simulink subsystem "VCM_main_djustablegain"  (R2021b)
settings: Solver=VariableStepAuto  StartTime=0.0  StopTime=10.0  RelTol=1e-3
undefined symbols (not defined in the file): df, dr, g, gear_f, gear_r, Iwf, Iwr, l, lf, M, Rwf, Rwr
libraries: simulink x43, dspstat3 x2, dspswit3 x1
(part 3 of 3)

== system VCM_main_djustablegain/VDC/Launch/max rpm ==
  Can Inv : Inport
  Bus Selector4 : BusSelector  OutputSignals=MC_11.MC1_Actual speed value in 1/rpm,MC_31.MC3_Actual speed value in 1/rpm,MC_21.MC2_Actual speed value in 1/rpm,MC_41.MC4_Actual speed value in 1/rpm
  Min : MinMax  Function=max  Inputs=4
  max rpm : Outport
  wires:
  Bus Selector4/2 -> Min/2  "<MC3_Actual speed value in 1/rpm>"
  Bus Selector4/3 -> Min/3  "<MC2_Actual speed value in 1/rpm>"
  Bus Selector4/1 -> Min/1  "<MC1_Actual speed value in 1/rpm>"
  Min/1 -> max rpm/1  "max rpm"
  Can Inv/1 -> Bus Selector4/1
  Bus Selector4/4 -> Min/4  "<MC4_Actual speed value in 1/rpm>"

== system VCM_main_djustablegain/VDC/Torque Front//rear distributor Main/Max Torque Limit ==
  note: MAXトルクオーバーしている分だけもう一方に振り直し
  Max Torque : Inport
  torque_front : Inport  Port=2
  torque_rear : Inport  Port=3
  Add10 : Sum  Inputs=-+
  Add11 : Sum
  Add4 : Sum  Inputs=+-
  Add7 : Sum  Inputs=+-
  Add8 : Sum
  Add9 : Sum  Inputs=+-
  Display : Display
  Display5 : Display
  Display6 : Display
  Saturation : Saturate  UpperLimit=inf  LowerLimit=0
  Saturation3 : Saturate  UpperLimit=inf  LowerLimit=0
  torque_front Out : Outport
  torque_rear Out : Outport  Port=2
  wires:
  Max Torque/1 -> Add9/2, Add4/2
  Add11/1 -> torque_rear Out/1
  Add7/1 -> Add11/2
  Add4/1 -> Saturation/1
  Add10/1 -> torque_front Out/1
  Add8/1 -> Add10/2
  torque_rear/1 -> Display6/1, Add7/1, Add4/1
  Add9/1 -> Saturation3/1
  torque_front/1 -> Display5/1, Add8/1, Add9/1
  Saturation3/1 -> Add10/1, Add11/1
  Saturation/1 -> Display/1, Add7/2, Add8/2

== system VCM_main_djustablegain/VDC/Torque Front//rear distributor Main/Min Torque Limit ==
  note: MINトルクオーバーしている分だけもう一方に振り直し
  Min Torque : Inport
  torque_front : Inport  Port=2
  torque_rear : Inport  Port=3
  Add10 : Sum  Inputs=-+
  Add11 : Sum
  Add4 : Sum  Inputs=+-
  Add7 : Sum  Inputs=+-
  Add8 : Sum
  Add9 : Sum  Inputs=+-
  Display{,1..2,5..6} (5 alike) : Display
  Gain : Gain  Gain=-1
  Saturation : Saturate  UpperLimit=0  LowerLimit=-inf
  Saturation3 : Saturate  UpperLimit=0  LowerLimit=-inf
  torque_rear Out : Outport
  torque_front Out : Outport  Port=2
  wires:
  Gain/1 -> Add9/2, Add4/2
  Min Torque/1 -> Gain/1
  Add11/1 -> torque_rear Out/1  "torque_rear"
  Add7/1 -> Add11/2, Display1/1
  Add4/1 -> Saturation/1
  Add10/1 -> torque_front Out/1  "torque_front"
  Add8/1 -> Add10/2
  torque_rear/1 -> Display6/1, Add7/1, Add4/1
  Add9/1 -> Saturation3/1
  torque_front/1 -> Display5/1, Add8/1, Add9/1
  Saturation3/1 -> Add10/1, Add11/1, Display2/1
  Saturation/1 -> Display/1, Add7/2, Add8/2

== system VCM_main_djustablegain/VDC/Torque Front//rear distributor Main/Saturation ==
  u : Inport
  Saturation Dynamic1 : simulink/Discontinuities/Saturation Dynamic  OutMin=[]  OutMax=[]  OutDataTypeStr=Inherit: Same as second input  OutDataType=fixdt(1, 16)  OutScaling=2^-10  DoSatur=off
  y : Outport
  wires:
  [MinTorque] -> Saturation Dynamic1/3
  u/1 -> Saturation Dynamic1/2
  Saturation Dynamic1/1 -> y/1
  [MaxTorque] -> Saturation Dynamic1/1

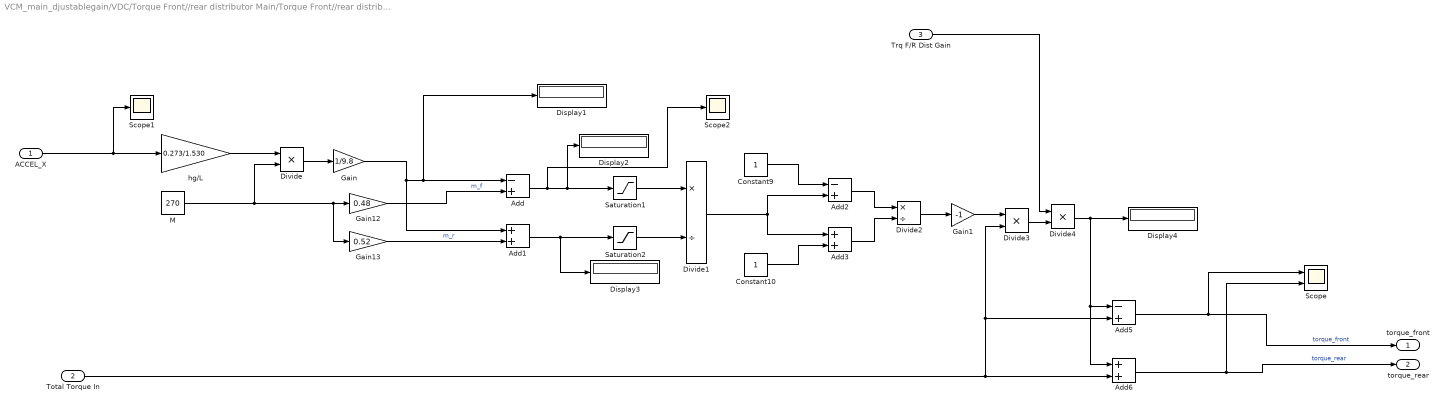
== system VCM_main_djustablegain/VDC/Torque Front//rear distributor Main/Torque Front//rear distributor  ==
  ACCEL_X : Inport
  Total Torque In : Inport  Port=2
  Trq F/R Dist Gain : Inport  Port=3
  Add : Sum  Inputs=-+
  Add1 : Sum
  Add2 : Sum  Inputs=-+
  Add3 : Sum
  Add5 : Sum  Inputs=-+
  Add6 : Sum
  Constant10 : Constant
  Constant9 : Constant
  Display{1..4} (4 alike) : Display
  Divide : Product  Inputs=**
  Divide1 : Product  Inputs=*/
  Divide2 : Product  Inputs=*/
  Divide3 : Product  Inputs=**
  Divide4 : Product  Inputs=**
  Gain : Gain  Gain=1/9.8
  Gain1 : Gain  Gain=-1
  Gain12 : Gain  Gain=0.48
  Gain13 : Gain  Gain=0.52
  M : Constant  Value=270
  Saturation1 : Saturate  UpperLimit=270  LowerLimit=10
  Saturation2 : Saturate  UpperLimit=270  LowerLimit=10
  Scope : Scope  NumInputPorts=2
  Scope1 : Scope
  Scope2 : Scope
  hg/L : Gain  Gain=0.273/1.530
  torque_front : Outport
  torque_rear : Outport  Port=2
  wires:
  Divide/1 -> Gain/1
  Total Torque In/1 -> Divide3/2, Add5/2, Add6/2
  Trq F/R Dist Gain/1 -> Divide4/1
  Divide3/1 -> Divide4/2
  Add5/1 -> torque_front/1, Scope/1  "torque_front"
  Add6/1 -> torque_rear/1, Scope/2  "torque_rear"
  Gain13/1 -> Add1/2  "m_r"
  Saturation1/1 -> Divide1/1
  Add/1 -> Saturation1/1, Display2/1, Scope2/1
  Gain/1 -> Add/1, Display1/1, Add1/1
  Add1/1 -> Saturation2/1, Display3/1
  ACCEL_X/1 -> hg/L/1, Scope1/1
  hg/L/1 -> Divide/1
  Constant10/1 -> Add3/2
  Gain1/1 -> Divide3/1
  Add2/1 -> Divide2/1
  Gain12/1 -> Add/2  "m_f"
  Divide2/1 -> Gain1/1
  Constant9/1 -> Add2/1
  Saturation2/1 -> Divide1/2
  Divide4/1 -> Display4/1, Add5/1, Add6/1
  Add3/1 -> Divide2/2
  Divide1/1 -> Add2/2, Add3/1
  M/1 -> Gain12/1, Gain13/1, Divide/2

== system VCM_main_djustablegain/VDC/Traction Control/Acc Estimater ==
  1/Gear{1..4} (4 alike) : Gain  Gain=gear_r
  Add : Sum  Inputs=++++
  EstLongAcc1 : Scope
  Gain : Gain  Gain=1/(M+2*Iwf/Rwf/Rwf+2*Iwr/Rwr/Rwr)
  Gain1 : Gain  Gain=1/g
  Moving Average : dspstat3/Moving Average  Method=Sliding window  ForgettingFactorPort=off  SpecifyWindowLength=on  WindowLength=10  ForgettingFactor=0.9  SimulateUsing=Code generation
  Rtire{1..4} (4 alike) : Gain  Gain=1/Rwf
  Saturation : Saturate  UpperLimit=1.3*g  LowerLimit=-1.3*g
  EstLongAcc : Outport
  wires:
  [FL_Torque] -> 1/Gear2/1
  Gain/1 -> Moving Average/1  "LongAcc"
  Rtire1/1 -> Add/1
  [RL_Torque] -> 1/Gear4/1
  Rtire3/1 -> Add/3
  1/Gear3/1 -> Rtire4/1
  [FR_Torque] -> 1/Gear1/1
  1/Gear2/1 -> Rtire1/1
  Saturation/1 -> EstLongAcc/1, Gain1/1  "LongAcc"
  Rtire2/1 -> Add/2
  Add/1 -> Gain/1
  1/Gear1/1 -> Rtire2/1
  Gain1/1 -> EstLongAcc1/1
  Rtire4/1 -> Add/4
  1/Gear4/1 -> Rtire3/1
  Moving Average/1 -> Saturation/1
  [RR_Torque] -> 1/Gear3/1

== system VCM_main_djustablegain/VDC/Traction Control/ActualSpeed ==
  Bus Creator : BusCreator  Inputs=4
  ActualSpeed : Outport
  wires:
  [RL_ActualSpeed] -> Bus Creator/3  "RL"
  [FR_ActualSpeed] -> Bus Creator/2  "FR"
  [FL_ActualSpeed] -> Bus Creator/1  "FL"
  [RR_ActualSpeed] -> Bus Creator/4  "RR"
  Bus Creator/1 -> ActualSpeed/1  "ActualSpeed"

== system VCM_main_djustablegain/VDC/Traction Control/Fx Estimater ==
  Bus Creator : BusCreator  Inputs=4
  EstFx : Scope
  FxEstimater : Subsystem
  FxEstimater1 : Subsystem
  FxEstimater2 : Subsystem
  FxEstimater3 : Subsystem
  Fx : Outport
  wires:
  FxEstimater1/1(Fx) -> Bus Creator/2  "FR"
  Bus Creator/1 -> Fx/1, EstFx/1  "Fx"
  FxEstimater3/1(Fx) -> Bus Creator/4  "RR"
  FxEstimater2/1(Fx) -> Bus Creator/3  "RL"
  FxEstimater/1(Fx) -> Bus Creator/1  "FL"
  [FL_Torque] -> FxEstimater/1(Torque)
  [FL_ActualSpeed] -> FxEstimater/2(ActualSpeed)
  [FR_ActualSpeed] -> FxEstimater1/2(ActualSpeed)
  [FR_Torque] -> FxEstimater1/1(Torque)
  [RR_Torque] -> FxEstimater3/1(Torque)
  [RR_ActualSpeed] -> FxEstimater3/2(ActualSpeed)
  [RL_ActualSpeed] -> FxEstimater2/2(ActualSpeed)
  [RL_Torque] -> FxEstimater2/1(Torque)

== system VCM_main_djustablegain/VDC/Traction Control/Load Estimater ==
  Long Acc : Inport
  Sensor : Inport  Port=2
  Steer : Inport  Port=3
  Bus Creator : BusCreator  Inputs=4
  Bus Selector : BusSelector  OutputSignals=CAN_from_IMU_139.VELOCITY_X
  Bus Selector1 : BusSelector  OutputSignals=CAN_from_IMU_121.ACCEL_Y
  Constant : Constant  Value=l
  Divide : Product  Inputs=*/
  Divide1 : Product  Inputs=*/
  EstAcc : Scope  NumInputPorts=2
  EstLoad : Scope
  FR Load Diff : Subsystem  ReferencedSubsystem=FR_Load_Diff
  Gain : Gain  Gain=1/(2*pi)
  Off : Gain  Gain=0
  Product : Product
  RL Load Diff : Subsystem  ReferencedSubsystem=RL_Load_Diff
  Load : Outport
  wires:
  Constant/1 -> Divide/1
  Divide/1 -> Divide1/2  "R"
  RL Load Diff/4 -> Bus Creator/4  "RR"
  Divide1/1 -> EstAcc/2
  Steer/1 -> Gain/1
  RL Load Diff/1 -> Bus Creator/1  "FL"
  FR Load Diff/1 -> RL Load Diff/1  "FrontLoad"
  Bus Selector1/1 -> Off/1  "<ACCEL_Y>"
  FR Load Diff/2 -> RL Load Diff/2  "RearLoad"
  RL Load Diff/2 -> Bus Creator/2  "FR"
  Long Acc/1 -> FR Load Diff/1, EstAcc/1
  RL Load Diff/3 -> Bus Creator/3  "RL"
  Gain/1 -> Divide/2
  Off/1 -> RL Load Diff/3
  Bus Creator/1 -> Load/1, EstLoad/1  "Load"
  Sensor/1 -> Bus Selector1/1, Bus Selector/1
  Bus Selector/1 -> Product/1, Product/2  "<VELOCITY_X>"
  Product/1 -> Divide1/1

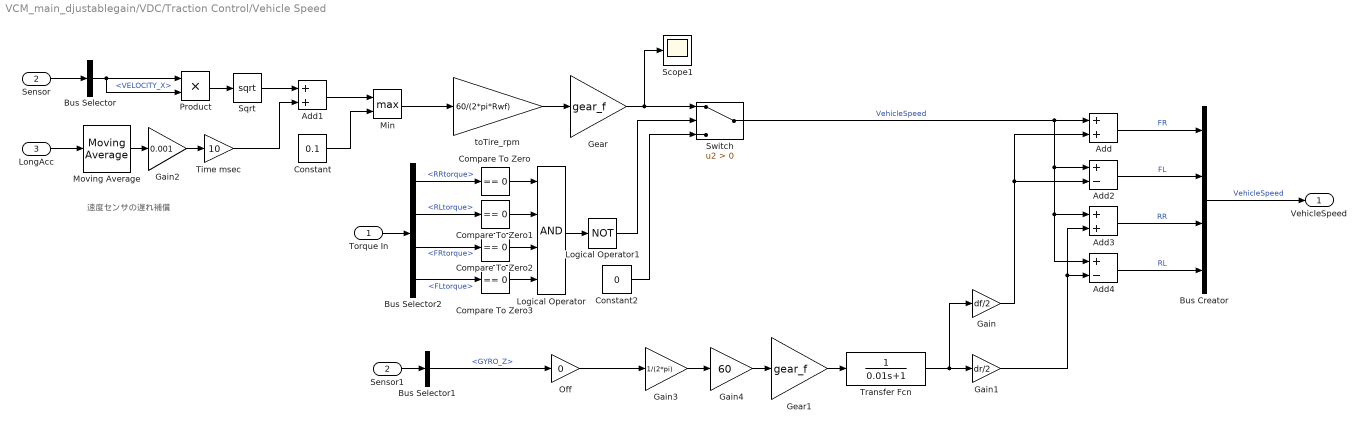
== system VCM_main_djustablegain/VDC/Traction Control/Vehicle Speed ==
  note: 速度センサの遅れ補償
  Torque In : Inport
  Sensor : Inport  Port=2
  LongAcc : Inport  Port=3
  Add : Sum
  Add1 : Sum
  Add2 : Sum  Inputs=+-
  Add3 : Sum
  Add4 : Sum  Inputs=+-
  Bus Creator : BusCreator  Inputs=4
  Bus Selector : BusSelector  OutputSignals=CAN_from_IMU_139.VELOCITY_X
  Bus Selector1 : BusSelector  OutputSignals=CAN_from_IMU_122.GYRO_Z
  Bus Selector2 : BusSelector  OutputSignals=RRtorque,RLtorque,FRtorque,FLtorque
  Compare To Zero{,1..3} (4 alike) : simulink/Logic and Bit Operations/Compare To Zero  relop===  OutDataTypeStr=boolean
  Constant : Constant  Value=0.1
  Constant2 : Constant  Value=0
  Gain : Gain  Gain=df/2
  Gain1 : Gain  Gain=dr/2
  Gain2 : Gain  Gain=0.001
  Gain3 : Gain  Gain=1/(2*pi)
  Gain4 : Gain  Gain=60
  Gear : Gain  Gain=gear_f
  Gear1 : Gain  Gain=gear_f
  Logical Operator : Logic  Inputs=4  AllPortsSameDT=off  OutDataTypeStr=boolean
  Logical Operator1 : Logic  Operator=NOT  AllPortsSameDT=off  OutDataTypeStr=boolean
  Min : MinMax  Function=max  Inputs=2
  Moving Average : dspstat3/Moving Average  Method=Sliding window  ForgettingFactorPort=off  SpecifyWindowLength=on  WindowLength=80  ForgettingFactor=0.9  SimulateUsing=Code generation
  Off : Gain  Gain=0
  Product : Product
  Scope1 : Scope
  Sensor1 : InportShadow  Port=2
  Sqrt : Sqrt  SaturateOnIntegerOverflow=on
  Switch : Switch  Criteria=u2 > Threshold
  Time msec : Gain  Gain=10
  Transfer Fcn : TransferFcn  Denominator=[0.01 1]
  toTire_rpm : Gain  Gain=60/(2*pi*Rwf)
  VehicleSpeed : Outport
  wires:
  Gain3/1 -> Gain4/1
  Bus Selector1/1 -> Off/1  "<GYRO_Z>"
  Product/1 -> Sqrt/1
  Transfer Fcn/1 -> Gain1/1, Gain/1
  Bus Selector/1 -> Product/1, Product/2  "<VELOCITY_X>"
  Switch/1 -> Add/1, Add2/1, Add4/1, Add3/1  "VehicleSpeed"
  Compare To Zero/1 -> Logical Operator/1
  Sensor/1 -> Bus Selector/1
  Bus Selector2/4 -> Compare To Zero3/1  "<FLtorque>"
  Compare To Zero2/1 -> Logical Operator/3
  Torque In/1 -> Bus Selector2/1
  LongAcc/1 -> Moving Average/1
  Sqrt/1 -> Add1/1
  Gear/1 -> Scope1/1, Switch/1
  toTire_rpm/1 -> Gear/1
  Gain1/1 -> Add3/2, Add4/2
  Logical Operator/1 -> Logical Operator1/1
  Add3/1 -> Bus Creator/3  "RR"
  Bus Selector2/1 -> Compare To Zero/1  "<RRtorque>"
  Logical Operator1/1 -> Switch/2
  Sensor1/1 -> Bus Selector1/1
  Compare To Zero3/1 -> Logical Operator/4
  Constant/1 -> Min/2
  Bus Selector2/2 -> Compare To Zero1/1  "<RLtorque>"
  Time msec/1 -> Add1/2
  Bus Selector2/3 -> Compare To Zero2/1  "<FRtorque>"
  Compare To Zero1/1 -> Logical Operator/2
  Off/1 -> Gain3/1
  Constant2/1 -> Switch/3
  Min/1 -> toTire_rpm/1
  Gain/1 -> Add/2, Add2/2
  Add1/1 -> Min/1
  Add2/1 -> Bus Creator/2  "FL"
  Moving Average/1 -> Gain2/1
  Add/1 -> Bus Creator/1  "FR"
  Add4/1 -> Bus Creator/4  "RL"
  Gain2/1 -> Time msec/1
  Gain4/1 -> Gear1/1
  Bus Creator/1 -> VehicleSpeed/1  "VehicleSpeed"
  Gear1/1 -> Transfer Fcn/1

== system VCM_main_djustablegain/VDC/VCM_Status/Sliprate ==
  from Sensor : Inport
  Bus Creator : BusCreator  Inputs=4
  Bus Selector4 : BusSelector  OutputSignals=CAN_from_IMU_139.VELOCITY_X
  Scope : Scope  NumInputPorts=4
  SlipRateClc FL : Subsystem  ReferencedSubsystem=SlipRateClc
  SlipRateClc FR : Subsystem  ReferencedSubsystem=SlipRateClc
  SlipRateClc RL : Subsystem  ReferencedSubsystem=SlipRateClc
  SlipRateClc RR : Subsystem  ReferencedSubsystem=SlipRateClc
  Tire rpm{,1..3} (4 alike) : Gain  Gain=1/gear_f
  to m/s{,1..3} (4 alike) : Gain  Gain=(2*pi*Rwf)/60
  Sliprate : Outport
  wires:
  to m/s1/1 -> SlipRateClc RR/1
  Tire rpm3/1 -> to m/s3/1
  SlipRateClc FR/1 -> Bus Creator/4, Scope/4  "FR"
  Bus Selector4/1 -> SlipRateClc FR/2, SlipRateClc RL/2, SlipRateClc RR/2, SlipRateClc FL/2  "<VELOCITY_X>"
  SlipRateClc RR/1 -> Bus Creator/2, Scope/2  "RR"
  SlipRateClc FL/1 -> Bus Creator/1, Scope/1  "FL"
  Bus Creator/1 -> Sliprate/1  "Sliprate"
  SlipRateClc RL/1 -> Bus Creator/3, Scope/3  "RL"
  Tire rpm1/1 -> to m/s1/1
  to m/s/1 -> SlipRateClc FL/1
  [FL_ActualSpeed] -> Tire rpm/1
  to m/s2/1 -> SlipRateClc RL/1
  Tire rpm/1 -> to m/s/1
  [RL_ActualSpeed] -> Tire rpm2/1
  [FR_ActualSpeed] -> Tire rpm3/1
  [RR_ActualSpeed] -> Tire rpm1/1
  to m/s3/1 -> SlipRateClc FR/1
  Tire rpm2/1 -> to m/s2/1
  from Sensor/1 -> Bus Selector4/1

== system VCM_main_djustablegain/VDC/VCM_Status/VCMStatus_bus ==
  In1 : Inport
  Bus Creator1 : BusCreator  Inputs=7
  Logical Operator1 : Logic  AllPortsSameDT=off  OutDataTypeStr=boolean
  VCMStatus : Outport
  wires:
  Bus Creator1/1 -> VCMStatus/1  "VCMStatus"
  In1/1 -> Logical Operator1/1
  [PowerLimitOn] -> Bus Creator1/7  "80kWOn"
  [TCOn] -> Bus Creator1/4  "TCOn"
  Logical Operator1/1 -> Bus Creator1/1  "VDCStatus"
  [VDCOn] -> Logical Operator1/2
  [DYCOn] -> Bus Creator1/6  "DYCOn"
  [ABSOn] -> Bus Creator1/5  "ABSOn"
  [BrakeOverRide] -> Bus Creator1/3  "BrakeOverRide"
  [APPS_SafetyError] -> Bus Creator1/2  "APPS_SafetyError"

== system VCM_main_djustablegain/Error display Box/Error Info/error memory MC1/Triggered Subsystem ==
  In1 : Inport
  Trigger : TriggerPort  VariantControl=Variant
  Delay : Delay  DelayLength=1  InitialCondition=0
  Delay1 : Delay  InitialCondition=0
  Out1 : Outport  VectorParamsAs1DForOutWhenUnconnected=off
  Out2 : Outport  Port=2  InitialOutput=[0]  VectorParamsAs1DForOutWhenUnconnected=off
  Out3 : Outport  Port=3  InitialOutput=[0]  VectorParamsAs1DForOutWhenUnconnected=off
  wires:
  Delay1/1 -> Out3/1
  Delay/1 -> Out2/1
  In1/1 -> Out1/1, Delay1/1, Delay/1

== system VCM_main_djustablegain/Error display Box/Error Info/error memory MC2/Triggered Subsystem ==
  In1 : Inport
  Trigger : TriggerPort  VariantControl=Variant
  Delay : Delay  DelayLength=1  InitialCondition=0
  Delay1 : Delay  InitialCondition=0
  Out1 : Outport  VectorParamsAs1DForOutWhenUnconnected=off
  Out2 : Outport  Port=2  InitialOutput=[0]  VectorParamsAs1DForOutWhenUnconnected=off
  Out3 : Outport  Port=3  InitialOutput=[0]  VectorParamsAs1DForOutWhenUnconnected=off
  wires:
  Delay1/1 -> Out3/1
  Delay/1 -> Out2/1
  In1/1 -> Out1/1, Delay1/1, Delay/1

== system VCM_main_djustablegain/Error display Box/Error Info/error memory MC3/Triggered Subsystem ==
  In1 : Inport
  Trigger : TriggerPort  VariantControl=Variant
  Delay : Delay  DelayLength=1  InitialCondition=0
  Delay1 : Delay  InitialCondition=0
  Out1 : Outport  VectorParamsAs1DForOutWhenUnconnected=off
  Out2 : Outport  Port=2  InitialOutput=[0]  VectorParamsAs1DForOutWhenUnconnected=off
  Out3 : Outport  Port=3  InitialOutput=[0]  VectorParamsAs1DForOutWhenUnconnected=off
  wires:
  Delay1/1 -> Out3/1
  Delay/1 -> Out2/1
  In1/1 -> Out1/1, Delay1/1, Delay/1

== system VCM_main_djustablegain/Error display Box/Error Info/error memory MC4/Triggered Subsystem ==
  In1 : Inport
  Trigger : TriggerPort  VariantControl=Variant
  Delay : Delay  DelayLength=1  InitialCondition=0
  Delay1 : Delay  InitialCondition=0
  Out1 : Outport  VectorParamsAs1DForOutWhenUnconnected=off
  Out2 : Outport  Port=2  InitialOutput=[0]  VectorParamsAs1DForOutWhenUnconnected=off
  Out3 : Outport  Port=3  InitialOutput=[0]  VectorParamsAs1DForOutWhenUnconnected=off
  wires:
  Delay1/1 -> Out3/1
  Delay/1 -> Out2/1
  In1/1 -> Out1/1, Delay1/1, Delay/1

== system VCM_main_djustablegain/Error display Box/Error Info1/error memory MC1/Triggered Subsystem ==
  In1 : Inport
  Trigger : TriggerPort  VariantControl=Variant
  Delay : Delay  DelayLength=1  InitialCondition=0
  Delay1 : Delay  InitialCondition=0
  Out1 : Outport  VectorParamsAs1DForOutWhenUnconnected=off
  Out2 : Outport  Port=2  InitialOutput=[0]  VectorParamsAs1DForOutWhenUnconnected=off
  Out3 : Outport  Port=3  InitialOutput=[0]  VectorParamsAs1DForOutWhenUnconnected=off
  wires:
  Delay1/1 -> Out3/1
  Delay/1 -> Out2/1
  In1/1 -> Out1/1, Delay/1, Delay1/1

== system VCM_main_djustablegain/Error display Box/Error Info1/error memory MC2/Triggered Subsystem ==
  In1 : Inport
  Trigger : TriggerPort  VariantControl=Variant
  Delay : Delay  DelayLength=1  InitialCondition=0
  Delay1 : Delay  InitialCondition=0
  Out1 : Outport  VectorParamsAs1DForOutWhenUnconnected=off
  Out2 : Outport  Port=2  InitialOutput=[0]  VectorParamsAs1DForOutWhenUnconnected=off
  Out3 : Outport  Port=3  InitialOutput=[0]  VectorParamsAs1DForOutWhenUnconnected=off
  wires:
  Delay1/1 -> Out3/1
  Delay/1 -> Out2/1
  In1/1 -> Out1/1, Delay/1, Delay1/1

== system VCM_main_djustablegain/Error display Box/Error Info1/error memory MC3/Triggered Subsystem ==
  In1 : Inport
  Trigger : TriggerPort  VariantControl=Variant
  Delay : Delay  DelayLength=1  InitialCondition=0
  Delay1 : Delay  InitialCondition=0
  Out1 : Outport  VectorParamsAs1DForOutWhenUnconnected=off
  Out2 : Outport  Port=2  InitialOutput=[0]  VectorParamsAs1DForOutWhenUnconnected=off
  Out3 : Outport  Port=3  InitialOutput=[0]  VectorParamsAs1DForOutWhenUnconnected=off
  wires:
  Delay1/1 -> Out3/1
  Delay/1 -> Out2/1
  In1/1 -> Out1/1, Delay/1, Delay1/1

== system VCM_main_djustablegain/Error display Box/Error Info1/error memory MC4/Triggered Subsystem ==
  In1 : Inport
  Trigger : TriggerPort  VariantControl=Variant
  Delay : Delay  DelayLength=1  InitialCondition=0
  Delay1 : Delay  InitialCondition=0
  Out1 : Outport  VectorParamsAs1DForOutWhenUnconnected=off
  Out2 : Outport  Port=2  InitialOutput=[0]  VectorParamsAs1DForOutWhenUnconnected=off
  Out3 : Outport  Port=3  InitialOutput=[0]  VectorParamsAs1DForOutWhenUnconnected=off
  wires:
  Delay1/1 -> Out3/1
  Delay/1 -> Out2/1
  In1/1 -> Out1/1, Delay/1, Delay1/1

== system VCM_main_djustablegain/Error display Box/Error Info2/error memory MC1/Triggered Subsystem ==
  In1 : Inport
  Trigger : TriggerPort  VariantControl=Variant
  Delay : Delay  DelayLength=1  InitialCondition=0
  Delay1 : Delay  InitialCondition=0
  Out1 : Outport  VectorParamsAs1DForOutWhenUnconnected=off
  Out2 : Outport  Port=2  InitialOutput=[0]  VectorParamsAs1DForOutWhenUnconnected=off
  Out3 : Outport  Port=3  InitialOutput=[0]  VectorParamsAs1DForOutWhenUnconnected=off
  wires:
  Delay1/1 -> Out3/1
  Delay/1 -> Out2/1
  In1/1 -> Out1/1, Delay/1, Delay1/1

== system VCM_main_djustablegain/Error display Box/Error Info2/error memory MC2/Triggered Subsystem ==
  In1 : Inport
  Trigger : TriggerPort  VariantControl=Variant
  Delay : Delay  DelayLength=1  InitialCondition=0
  Delay1 : Delay  InitialCondition=0
  Out1 : Outport  VectorParamsAs1DForOutWhenUnconnected=off
  Out2 : Outport  Port=2  InitialOutput=[0]  VectorParamsAs1DForOutWhenUnconnected=off
  Out3 : Outport  Port=3  InitialOutput=[0]  VectorParamsAs1DForOutWhenUnconnected=off
  wires:
  Delay1/1 -> Out3/1
  Delay/1 -> Out2/1
  In1/1 -> Out1/1, Delay/1, Delay1/1

== system VCM_main_djustablegain/Error display Box/Error Info2/error memory MC3/Triggered Subsystem ==
  In1 : Inport
  Trigger : TriggerPort  VariantControl=Variant
  Delay : Delay  DelayLength=1  InitialCondition=0
  Delay1 : Delay  InitialCondition=0
  Out1 : Outport  VectorParamsAs1DForOutWhenUnconnected=off
  Out2 : Outport  Port=2  InitialOutput=[0]  VectorParamsAs1DForOutWhenUnconnected=off
  Out3 : Outport  Port=3  InitialOutput=[0]  VectorParamsAs1DForOutWhenUnconnected=off
  wires:
  Delay1/1 -> Out3/1
  Delay/1 -> Out2/1
  In1/1 -> Out1/1, Delay/1, Delay1/1

== system VCM_main_djustablegain/Error display Box/Error Info2/error memory MC4/Triggered Subsystem ==
  In1 : Inport
  Trigger : TriggerPort  VariantControl=Variant
  Delay : Delay  DelayLength=1  InitialCondition=0
  Delay1 : Delay  InitialCondition=0
  Out1 : Outport  VectorParamsAs1DForOutWhenUnconnected=off
  Out2 : Outport  Port=2  InitialOutput=[0]  VectorParamsAs1DForOutWhenUnconnected=off
  Out3 : Outport  Port=3  InitialOutput=[0]  VectorParamsAs1DForOutWhenUnconnected=off
  wires:
  Delay1/1 -> Out3/1
  Delay/1 -> Out2/1
  In1/1 -> Out1/1, Delay/1, Delay1/1

== system VCM_main_djustablegain/Error display Box/Error Info3/error memory MC1/Triggered Subsystem ==
  In1 : Inport
  Trigger : TriggerPort  VariantControl=Variant
  Delay : Delay  DelayLength=1  InitialCondition=0
  Delay1 : Delay  InitialCondition=0
  Out1 : Outport  VectorParamsAs1DForOutWhenUnconnected=off
  Out2 : Outport  Port=2  InitialOutput=[0]  VectorParamsAs1DForOutWhenUnconnected=off
  Out3 : Outport  Port=3  InitialOutput=[0]  VectorParamsAs1DForOutWhenUnconnected=off
  wires:
  Delay1/1 -> Out3/1
  Delay/1 -> Out2/1
  In1/1 -> Out1/1, Delay/1, Delay1/1

== system VCM_main_djustablegain/Error display Box/Error Info3/error memory MC2/Triggered Subsystem ==
  In1 : Inport
  Trigger : TriggerPort  VariantControl=Variant
  Delay : Delay  DelayLength=1  InitialCondition=0
  Delay1 : Delay  InitialCondition=0
  Out1 : Outport  VectorParamsAs1DForOutWhenUnconnected=off
  Out2 : Outport  Port=2  InitialOutput=[0]  VectorParamsAs1DForOutWhenUnconnected=off
  Out3 : Outport  Port=3  InitialOutput=[0]  VectorParamsAs1DForOutWhenUnconnected=off
  wires:
  Delay1/1 -> Out3/1
  Delay/1 -> Out2/1
  In1/1 -> Out1/1, Delay/1, Delay1/1

== system VCM_main_djustablegain/Error display Box/Error Info3/error memory MC3/Triggered Subsystem ==
  In1 : Inport
  Trigger : TriggerPort  VariantControl=Variant
  Delay : Delay  DelayLength=1  InitialCondition=0
  Delay1 : Delay  InitialCondition=0
  Out1 : Outport  VectorParamsAs1DForOutWhenUnconnected=off
  Out2 : Outport  Port=2  InitialOutput=[0]  VectorParamsAs1DForOutWhenUnconnected=off
  Out3 : Outport  Port=3  InitialOutput=[0]  VectorParamsAs1DForOutWhenUnconnected=off
  wires:
  Delay1/1 -> Out3/1
  Delay/1 -> Out2/1
  In1/1 -> Out1/1, Delay/1, Delay1/1

== system VCM_main_djustablegain/Error display Box/Error Info3/error memory MC4/Triggered Subsystem ==
  In1 : Inport
  Trigger : TriggerPort  VariantControl=Variant
  Delay : Delay  DelayLength=1  InitialCondition=0
  Delay1 : Delay  InitialCondition=0
  Out1 : Outport  VectorParamsAs1DForOutWhenUnconnected=off
  Out2 : Outport  Port=2  InitialOutput=[0]  VectorParamsAs1DForOutWhenUnconnected=off
  Out3 : Outport  Port=3  InitialOutput=[0]  VectorParamsAs1DForOutWhenUnconnected=off
  wires:
  Delay1/1 -> Out3/1
  Delay/1 -> Out2/1
  In1/1 -> Out1/1, Delay/1, Delay1/1

== system VCM_main_djustablegain/VDC/80kw_limitation/Power Limit_last/FeedBack ==
  Torque : Inport
  FB : Inport  Port=2
  Add : Sum
  Bus Selector3 : BusSelector  OutputSignals=torque
  FB Torque : Outport
  wires:
  Torque/1 -> Bus Selector3/1
  Add/1 -> FB Torque/1
  FB/1 -> Add/2
  Bus Selector3/1 -> Add/1  "<torque>"

== system VCM_main_djustablegain/VDC/80kw_limitation/Power Limit_last/FeedBack and Switch ==
  LimitTorque : Inport
  Torque : Inport  Port=2
  Bus Selector5 : BusSelector  OutputSignals=torque
  Max : MinMax  Function=max  Inputs=2
  Min : MinMax  Inputs=2
  Saturation Dynamic : simulink/Discontinuities/Saturation Dynamic  OutMin=[]  OutMax=[]  OutDataTypeStr=Inherit: Same as second input  OutDataType=fixdt(1, 16)  OutScaling=2^-10  DoSatur=off
  Switch : Switch  Criteria=u2 > Threshold
  Switch1 : Switch  Criteria=u2 > Threshold
  trq : Outport
  wires:
  [MinTorque] -> Saturation Dynamic/3
  Saturation Dynamic/1 -> trq/1
  Switch1/1 -> Saturation Dynamic/1  "torque"
  [PowerLimitOn] -> Switch1/2
  Torque/1 -> Bus Selector5/1
  Switch/1 -> Switch1/1  "torque"
  Min/1 -> Switch/1
  Max/1 -> Switch/3
  Bus Selector5/1 -> Min/1, Switch/2, Max/2, Switch1/3, Saturation Dynamic/2  "<torque>"
  LimitTorque/1 -> Min/2, Max/1

== system VCM_main_djustablegain/VDC/80kw_limitation/Power Limit_last/FeedBack and Switch1 ==
  LimitTorque : Inport
  Torque : Inport  Port=2
  Bus Selector5 : BusSelector  OutputSignals=torque
  Max : MinMax  Function=max  Inputs=2
  Min : MinMax  Inputs=2
  Saturation Dynamic : simulink/Discontinuities/Saturation Dynamic  OutMin=[]  OutMax=[]  OutDataTypeStr=Inherit: Same as second input  OutDataType=fixdt(1, 16)  OutScaling=2^-10  DoSatur=off
  Switch : Switch  Criteria=u2 > Threshold
  Switch1 : Switch  Criteria=u2 > Threshold
  trq : Outport
  wires:
  LimitTorque/1 -> Max/1, Min/2
  Bus Selector5/1 -> Saturation Dynamic/2, Switch1/3, Max/2, Switch/2, Min/1  "<torque>"
  Max/1 -> Switch/3
  Min/1 -> Switch/1
  Switch/1 -> Switch1/1  "torque"
  Torque/1 -> Bus Selector5/1
  [PowerLimitOn] -> Switch1/2
  Switch1/1 -> Saturation Dynamic/1  "torque"
  Saturation Dynamic/1 -> trq/1
  [MinTorque] -> Saturation Dynamic/3

== system VCM_main_djustablegain/VDC/80kw_limitation/Power Limit_last/FeedBack and Switch2 ==
  LimitTorque : Inport
  Torque : Inport  Port=2
  Bus Selector5 : BusSelector  OutputSignals=torque
  Max : MinMax  Function=max  Inputs=2
  Min : MinMax  Inputs=2
  Saturation Dynamic : simulink/Discontinuities/Saturation Dynamic  OutMin=[]  OutMax=[]  OutDataTypeStr=Inherit: Same as second input  OutDataType=fixdt(1, 16)  OutScaling=2^-10  DoSatur=off
  Switch : Switch  Criteria=u2 > Threshold
  Switch1 : Switch  Criteria=u2 > Threshold
  trq : Outport
  wires:
  [MinTorque] -> Saturation Dynamic/3
  Saturation Dynamic/1 -> trq/1
  Switch1/1 -> Saturation Dynamic/1  "torque"
  [PowerLimitOn] -> Switch1/2
  Torque/1 -> Bus Selector5/1
  Switch/1 -> Switch1/1  "torque"
  Min/1 -> Switch/1
  Max/1 -> Switch/3
  Bus Selector5/1 -> Min/1, Switch/2, Max/2, Switch1/3, Saturation Dynamic/2  "<torque>"
  LimitTorque/1 -> Min/2, Max/1

== system VCM_main_djustablegain/VDC/80kw_limitation/Power Limit_last/FeedBack and Switch3 ==
  LimitTorque : Inport
  Torque : Inport  Port=2
  Bus Selector5 : BusSelector  OutputSignals=torque
  Max : MinMax  Function=max  Inputs=2
  Min : MinMax  Inputs=2
  Saturation Dynamic : simulink/Discontinuities/Saturation Dynamic  OutMin=[]  OutMax=[]  OutDataTypeStr=Inherit: Same as second input  OutDataType=fixdt(1, 16)  OutScaling=2^-10  DoSatur=off
  Switch : Switch  Criteria=u2 > Threshold
  Switch1 : Switch  Criteria=u2 > Threshold
  trq : Outport
  wires:
  LimitTorque/1 -> Max/1, Min/2
  Bus Selector5/1 -> Saturation Dynamic/2, Switch1/3, Max/2, Switch/2, Min/1  "<torque>"
  Max/1 -> Switch/3
  Min/1 -> Switch/1
  Switch/1 -> Switch1/1  "torque"
  Torque/1 -> Bus Selector5/1
  [PowerLimitOn] -> Switch1/2
  Switch1/1 -> Saturation Dynamic/1  "torque"
  Saturation Dynamic/1 -> trq/1
  [MinTorque] -> Saturation Dynamic/3

== system VCM_main_djustablegain/VDC/80kw_limitation/Power Limit_last/FeedBack1 ==
  Torque : Inport
  FB : Inport  Port=2
  Add : Sum
  Bus Selector3 : BusSelector  OutputSignals=torque
  FB Torque : Outport
  wires:
  Bus Selector3/1 -> Add/1  "<torque>"
  FB/1 -> Add/2
  Add/1 -> FB Torque/1
  Torque/1 -> Bus Selector3/1

== system VCM_main_djustablegain/VDC/80kw_limitation/Power Limit_last/FeedBack2 ==
  Torque : Inport
  FB : Inport  Port=2
  Add : Sum
  Bus Selector3 : BusSelector  OutputSignals=torque
  FB Torque : Outport
  wires:
  Torque/1 -> Bus Selector3/1
  Add/1 -> FB Torque/1
  FB/1 -> Add/2
  Bus Selector3/1 -> Add/1  "<torque>"

== system VCM_main_djustablegain/VDC/80kw_limitation/Power Limit_last/FeedBack3 ==
  Torque : Inport
  FB : Inport  Port=2
  Add : Sum
  Bus Selector3 : BusSelector  OutputSignals=torque
  FB Torque : Outport
  wires:
  Bus Selector3/1 -> Add/1  "<torque>"
  FB/1 -> Add/2
  Add/1 -> FB Torque/1
  Torque/1 -> Bus Selector3/1

== system VCM_main_djustablegain/VDC/DYC/DYC main/Velocity Clc ==
  Sensor : Inport
  Add : Sum
  Bus Selector : BusSelector  OutputSignals=CAN_from_IMU_139.VELOCITY_X,CAN_from_IMU_139.VELOCITY_Y
  Sqrt : Sqrt  SaturateOnIntegerOverflow=on
  Square1 : Math  Operator=square  SaturateOnIntegerOverflow=on
  Square2 : Math  Operator=square  SaturateOnIntegerOverflow=on
  Transfer Fcn : TransferFcn  Denominator=[0.03 1]
  v [m/s] : Outport
  wires:
  Sqrt/1 -> Transfer Fcn/1  "v [m/s]"
  Transfer Fcn/1 -> v [m/s]/1  "v [m/s]"
  Square2/1 -> Add/2
  Sensor/1 -> Bus Selector/1
  Square1/1 -> Add/1
  Add/1 -> Sqrt/1
  Bus Selector/1 -> Square1/1  "<VELOCITY_X>"
  Bus Selector/2 -> Square2/1  "<VELOCITY_Y>"

== system VCM_main_djustablegain/VDC/Traction Control/Fx Estimater/FxEstimater ==
  Torque : Inport
  ActualSpeed : Inport  Port=2
  Add4 : Sum  Inputs=+-
  Discrete Derivative : simulink/Discrete/Discrete Derivative  gainval=1.0  ICPrevScaledInput=0.0  OutMin=[]  OutMax=[]  OutDataType=fixdt(1, 16)  OutScaling=2^-10  DoSatur=off
  Gain : Gain  Gain=gear_f
  Gain1 : Gain  Gain=1/60
  Gain2 : Gain  Gain=2*pi
  Gain3 : Gain  Gain=1/gear_f
  Gain4 : Gain  Gain=Iwf
  Gain5 : Gain  Gain=1/Rwf
  Fx : Outport
  wires:
  Gain1/1 -> Gain2/1
  Gain2/1 -> Discrete Derivative/1
  Torque/1 -> Gain/1
  Discrete Derivative/1 -> Gain4/1
  Gain/1 -> Add4/1
  Add4/1 -> Gain5/1
  Gain5/1 -> Fx/1
  Gain4/1 -> Add4/2
  ActualSpeed/1 -> Gain3/1
  Gain3/1 -> Gain1/1

== system VCM_main_djustablegain/VDC/Traction Control/Fx Estimater/FxEstimater1 ==
  Torque : Inport
  ActualSpeed : Inport  Port=2
  Add4 : Sum  Inputs=+-
  Discrete Derivative : simulink/Discrete/Discrete Derivative  gainval=1.0  ICPrevScaledInput=0.0  OutMin=[]  OutMax=[]  OutDataType=fixdt(1, 16)  OutScaling=2^-10  DoSatur=off
  Gain : Gain  Gain=gear_f
  Gain1 : Gain  Gain=1/60
  Gain2 : Gain  Gain=2*pi
  Gain3 : Gain  Gain=1/gear_f
  Gain4 : Gain  Gain=Iwf
  Gain5 : Gain  Gain=1/Rwf
  Fx : Outport
  wires:
  Gain3/1 -> Gain1/1
  ActualSpeed/1 -> Gain3/1
  Gain4/1 -> Add4/2
  Gain5/1 -> Fx/1
  Add4/1 -> Gain5/1
  Gain/1 -> Add4/1
  Discrete Derivative/1 -> Gain4/1
  Torque/1 -> Gain/1
  Gain2/1 -> Discrete Derivative/1
  Gain1/1 -> Gain2/1

== system VCM_main_djustablegain/VDC/Traction Control/Fx Estimater/FxEstimater2 ==
  Torque : Inport
  ActualSpeed : Inport  Port=2
  Add4 : Sum  Inputs=+-
  Discrete Derivative : simulink/Discrete/Discrete Derivative  gainval=1.0  ICPrevScaledInput=0.0  OutMin=[]  OutMax=[]  OutDataType=fixdt(1, 16)  OutScaling=2^-10  DoSatur=off
  Gain : Gain  Gain=gear_f
  Gain1 : Gain  Gain=1/60
  Gain2 : Gain  Gain=2*pi
  Gain3 : Gain  Gain=1/gear_f
  Gain4 : Gain  Gain=Iwf
  Gain5 : Gain  Gain=1/Rwf
  Fx : Outport
  wires:
  Gain1/1 -> Gain2/1
  Gain2/1 -> Discrete Derivative/1
  Torque/1 -> Gain/1
  Discrete Derivative/1 -> Gain4/1
  Gain/1 -> Add4/1
  Add4/1 -> Gain5/1
  Gain5/1 -> Fx/1
  Gain4/1 -> Add4/2
  ActualSpeed/1 -> Gain3/1
  Gain3/1 -> Gain1/1

== system VCM_main_djustablegain/VDC/Traction Control/Fx Estimater/FxEstimater3 ==
  Torque : Inport
  ActualSpeed : Inport  Port=2
  Add4 : Sum  Inputs=+-
  Discrete Derivative : simulink/Discrete/Discrete Derivative  gainval=1.0  ICPrevScaledInput=0.0  OutMin=[]  OutMax=[]  OutDataType=fixdt(1, 16)  OutScaling=2^-10  DoSatur=off
  Gain : Gain  Gain=gear_f
  Gain1 : Gain  Gain=1/60
  Gain2 : Gain  Gain=2*pi
  Gain3 : Gain  Gain=1/gear_f
  Gain4 : Gain  Gain=Iwf
  Gain5 : Gain  Gain=1/Rwf
  Fx : Outport
  wires:
  Gain3/1 -> Gain1/1
  ActualSpeed/1 -> Gain3/1
  Gain4/1 -> Add4/2
  Gain5/1 -> Fx/1
  Add4/1 -> Gain5/1
  Gain/1 -> Add4/1
  Discrete Derivative/1 -> Gain4/1
  Torque/1 -> Gain/1
  Gain2/1 -> Discrete Derivative/1
  Gain1/1 -> Gain2/1

== matlab function VCM_main_djustablegain/TrqClc ==
  data: MaxTorque input; Trq output; CoastTorque input; TorqueZeroPosi input; APPS input; APPS output
function [Trq, APPS] = fcn(MaxTorque, CoastTorque, TorqueZeroPosi, APPS)
    % Linear
    if APPS>=TorqueZeroPosi
        Trq=MaxTorque*(APPS-TorqueZeroPosi)/(1-TorqueZeroPosi);
    else
        Trq=-CoastTorque*(APPS-0)/(TorqueZeroPosi-0);
    end

    % A Curve
%     X=10;
%     if APPS>=Free
%         Trq=Max*(X^((APPS-Free)/(1-Free))-1)/(X-1);
%     else
%         Trq=0;
%     end
end

== matlab function VCM_main_djustablegain/VDC/DYC/DYC main/Target Moment ==
  data: Km input; M output; K0 input; V input; V0 input; delta input
function M = fcn(Km, K0, V, V0, delta)
    if V<3/3.6
        M=0;
    else
        M=Km*(1+(K0/Km-1)*exp(-V/V0))*delta;
    end
end

== matlab function VCM_main_djustablegain/VDC/DYC/DYC main/DYC Trq ==
  data: RR output; RL output; FR output; TrqF input; TrqR input; KF input; KR input; M input; FL output; delta input; lf parameter; df parameter
function [RR, RL, FR, FL] = fcn(TrqF, TrqR, KF, KR, M, delta, lf, df)
    FL=(1+2*lf/df*tan(delta))*TrqF-(KF*M)/(df*cos(delta));
    FR=(1-2*lf/df*tan(delta))*TrqF+(KF*M)/(df*cos(delta));
    RL=TrqR-(KR*M)/df;
    RR=TrqR+(KR*M)/df;
end

== stateflow chart VCM_main_djustablegain/VDC/Launch/Chart ==
  state Base
    entry:
    LaunchTorqueLimit = MaxTorqueLimit;
    LaunchLED = 0;
  state OFF
    entry:
    LaunchTorqueLimit = 0;
  state LaunchReady
    entry:
    LaunchTorqueLimit = MaxTorqueLimit;
  state LaunchReady_BrakeON
    entry:
    LaunchTorqueLimit = 0;
    LaunchLED = 1;
  state LaunchReady_BrakeOff
    entry:
    LaunchTorqueLimit = 0;
    state LaunchLEDon
      entry:
      LaunchLED = 1;
    state LaunchLEDoff
      entry:
      LaunchLED = 0;
    (default) -> LaunchLEDon
    LaunchLEDoff -> LaunchLEDon : after(0.2,sec)
    LaunchLEDon -> LaunchLEDoff : after(0.2,sec)
  state LaunchGearProtection
    entry:
    LaunchTorqueLimit = GearProtectionTorqueLimit;
    LaunchLED = 1;
  (default) -> Base
  OFF -> Base : [Torque< 0.5]
  LaunchGearProtection -> Base : after(GearProtectionTime,sec)
  (junction 24) -> OFF
  Base -> LaunchReady : [LaunchSW == 1 & BrakeSW == 1 & rpm < 10 & Torque < 0.3]
  LaunchReady -> (junction 24) [order 2] : [LaunchSW == 0]
  (junction 17) -> (junction 24)
  LaunchReady -> LaunchReady_BrakeON [order 1] : after(2,sec)[BrakeSW == 1]
  LaunchReady_BrakeON -> (junction 17) [order 1] : [LaunchSW == 0]
  LaunchReady_BrakeON -> LaunchReady_BrakeOff [order 2] : after(1,sec)[BrakeSW == 0 & Torque > 5 ]
  LaunchReady_BrakeOff -> LaunchReady_BrakeON [order 1] : [Torque < 4 | BrakeSW == 1]
  LaunchReady_BrakeOff -> LaunchGearProtection [order 2] : [LaunchSW == 0]
  data: LaunchSW input; BrakeSW input; rpm input; Torque input; MaxTorqueLimit input; GearProtectionTorqueLimit input; GearProtectionTime input; LaunchLED output; LaunchTorqueLimit output
